simulink model "RTForwardVehicleSensorFusionHost"  (R2022a)
settings: Solver=FixedStepAuto  StartTime=0.0  StopTime=scenario.StopTime  RelTol=1e-3
PostLoadFcn:
  | helperSLForwardVehicleSensorFusionHostSetup
values from neighbouring files (symbols this model uses):
  camera = cameraParams(egoVehicle)    [helperSLForwardVehicleSensorFusionHostSetup.m]
  vehSim3D = repmat(     struct(         'Length', 0,         'RearOverhang', 0,         'InitialPos',[0 0 0],         'InitialRot',[0 0 0]),     numVehicles,1)    [helperSLForwardVehicleSensorFusionHostSetup.m]
undefined symbols (not defined in the file or in its folder): maxNumRadarDets, maxNumTracks, maxNumVisionDets, Ts
libraries: drivingscenarioandsensors x8, sim3dautolib x6, slrealtimeiplib x3, slrealtimeutilitieslib x3, simulink x1, sim3dprobsensorlib x1, sim3dlib x1, drivingsim3d x1
CloseFcn:
  | helperSLForwardVehicleSensorFusionHostCleanUp
settings Model: SILPILSystemUnderTest=refmodels  PacingRate=0.050000  Creator=The MathWorks, Inc.  LastModifiedBy=The MathWorks, Inc.
settings SolverCC: AlgebraicLoopSolver=TrustRegion  MaxZcPerStep=1
settings DataIOCC: SaveOutput=off  SaveTime=off  ReturnWorkspaceOutputs=off
settings OptimizationCC: ZeroExternalMemoryAtStartup=off  ZeroInternalMemoryAtStartup=off
settings DebuggingCC: ParameterPrecisionLossMsg=none  UnconnectedInputMsg=warning  UnconnectedOutputMsg=warning  UnconnectedLineMsg=warning  PregeneratedLibrarySubsystemCodeDiagnostic=none  SFMachineParentedDataDiag=warning  ArithmeticOperatorsInVariantConditions=warning
settings HardwareCC: ProdLongLongMode=on
settings SFSimCC: SimUseLocalCustomCode=off  SimTargetLang=C++
settings RTWCC: RTWUseLocalCustomCode=off  TargetLang=C++  DLArmComputeVersion=19.05
settings GRTTargetCC: TargetLangStandard=C++03 (ISO)  CodeInterfacePackaging=C++ class  RTWCAPISignals=on
settings ConfigComp: CovScope=ReferencedModels  CovIncludeTopModel=off

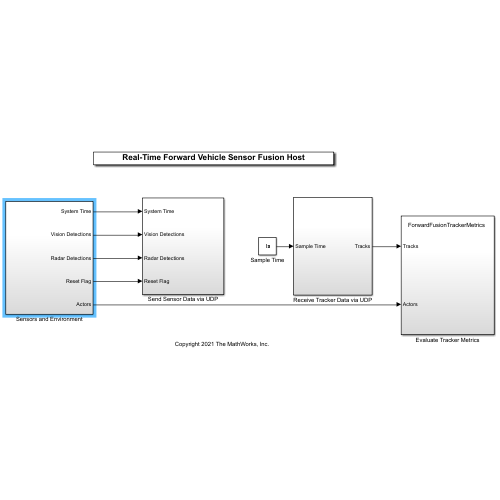
[thumbnail: Simulink's stored preview of the top-level diagram]
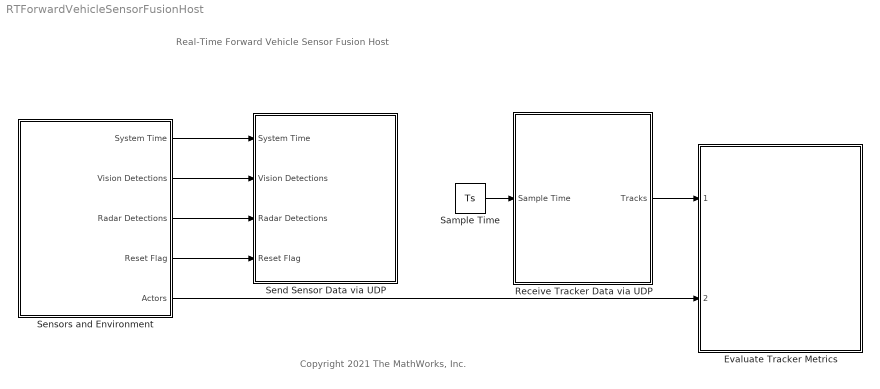
== system RTForwardVehicleSensorFusionHost ==
  note: Real-Time Forward Vehicle Sensor Fusion Host
  note: Copyright 2021 The MathWorks, Inc.
  Evaluate Tracker Metrics : Subsystem  ReferencedSubsystem=ForwardFusionTrackerMetrics
  Receive Tracker Data via UDP : Subsystem
  Sample Time : Constant  Value=Ts  SampleTime=Ts
  Send Sensor Data via UDP : Subsystem
  Sensors and Environment : Subsystem  VariantControl=1
  wires:
  Sensors and Environment/5(Actors) -> Evaluate Tracker Metrics/2
  Receive Tracker Data via UDP/1(Tracks) -> Evaluate Tracker Metrics/1
  Sensors and Environment/2(Vision Detections) -> Send Sensor Data via UDP/2(Vision Detections)
  Sensors and Environment/3(Radar Detections) -> Send Sensor Data via UDP/3(Radar Detections)
  Sensors and Environment/1(System Time) -> Send Sensor Data via UDP/1(System Time)
  Sample Time/1 -> Receive Tracker Data via UDP/1(Sample Time)
  Sensors and Environment/4(Reset Flag) -> Send Sensor Data via UDP/4(Reset Flag)

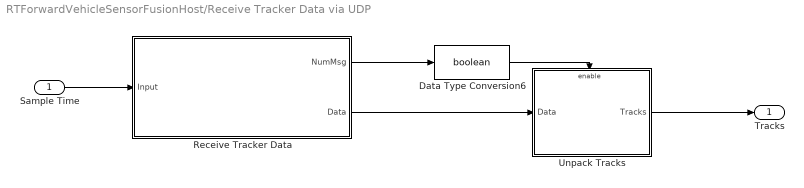
== system RTForwardVehicleSensorFusionHost/Receive Tracker Data via UDP ==
  Sample Time : Inport
  Data Type Conversion6 : DataTypeConversion  OutDataTypeStr=boolean  SaturateOnIntegerOverflow=off  RndMeth=Floor
  Receive Tracker Data : Subsystem
  Unpack Tracks : Subsystem
  Tracks : Outport
  wires:
  Data Type Conversion6/1 -> Unpack Tracks/Enable
  Receive Tracker Data/1(NumMsg) -> Data Type Conversion6/1
  Unpack Tracks/1(Tracks) -> Tracks/1
  Receive Tracker Data/2(Data) -> Unpack Tracks/1(Data)
  Sample Time/1 -> Receive Tracker Data/1(Input)

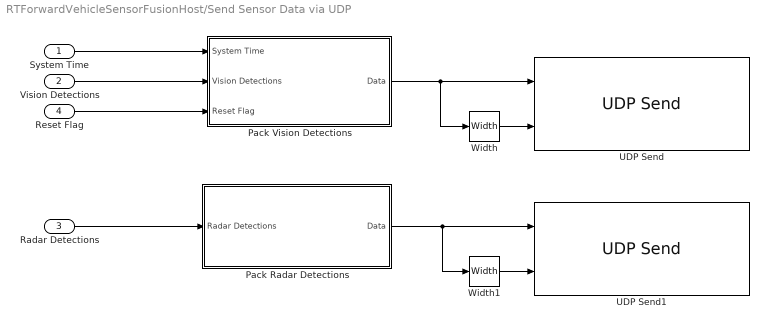
== system RTForwardVehicleSensorFusionHost/Send Sensor Data via UDP ==
  System Time : Inport
  Vision Detections : Inport  Port=2
  Radar Detections : Inport  Port=3
  Reset Flag : Inport  Port=4
  Pack Radar Detections : Subsystem
  Pack Vision Detections : Subsystem
  UDP Send : slrealtimeiplib/UDP Send  useHostTargetConn=on  toAddress=10.1.10.17  toPort=8001  sampleTime=-1  enableMessage=off  ipAddress=10.1.10.16  localPort=-1
      settings: SourceProductBaseCode=XP
  UDP Send1 : slrealtimeiplib/UDP Send  useHostTargetConn=on  toAddress=10.1.10.17  toPort=8002  sampleTime=-1  enableMessage=off  ipAddress=10.1.10.16  localPort=-1
      settings: SourceProductBaseCode=XP
  Width : Width
  Width1 : Width
  wires:
  Width/1 -> UDP Send/2
  Width1/1 -> UDP Send1/2
  Pack Vision Detections/1(Data) -> Width/1, UDP Send/1
  System Time/1 -> Pack Vision Detections/1(System Time)
  Vision Detections/1 -> Pack Vision Detections/2(Vision Detections)
  Reset Flag/1 -> Pack Vision Detections/3(Reset Flag)
  Pack Radar Detections/1(Data) -> Width1/1, UDP Send1/1
  Radar Detections/1 -> Pack Radar Detections/1(Radar Detections)

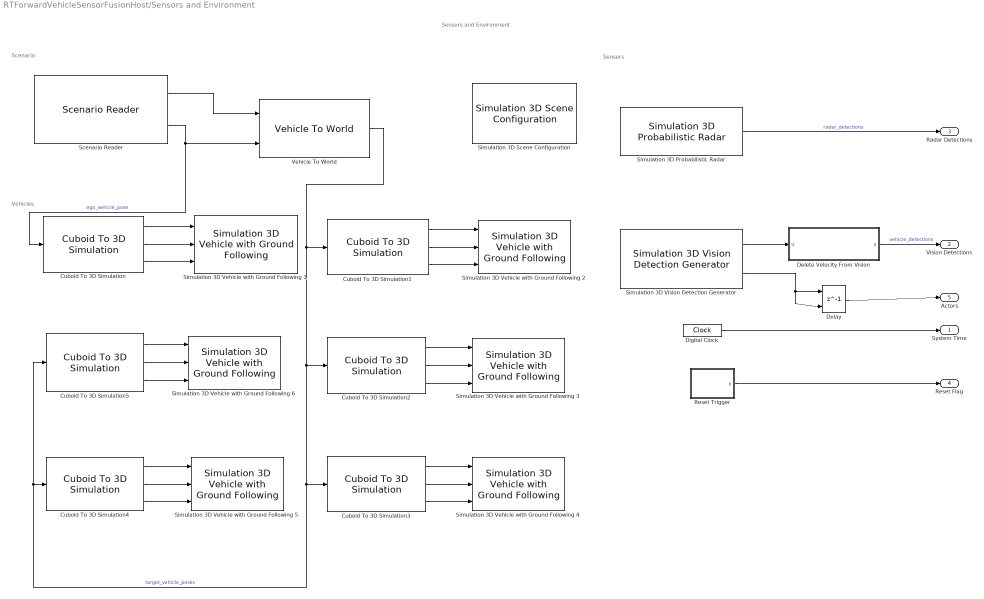
== system RTForwardVehicleSensorFusionHost/Sensors and Environment ==
  note: Sensors
  note: Sensors and Environment
  note: Scenario
  note: Vehicles
  Cuboid To 3D Simulation : drivingscenarioandsensors/Cuboid To 3D Simulation  SpecifyActorID=off  ActorIDToConvert=1  SimulateUsing=Interpreted execution
      settings: SourceProductBaseCode=DR
  Cuboid To 3D Simulation1 : drivingscenarioandsensors/Cuboid To 3D Simulation  SpecifyActorID=on  ActorIDToConvert=2  SimulateUsing=Interpreted execution
      settings: SourceProductBaseCode=DR
  Cuboid To 3D Simulation2 : drivingscenarioandsensors/Cuboid To 3D Simulation  SpecifyActorID=on  ActorIDToConvert=3  SimulateUsing=Interpreted execution
      settings: SourceProductBaseCode=DR
  Cuboid To 3D Simulation3 : drivingscenarioandsensors/Cuboid To 3D Simulation  SpecifyActorID=on  ActorIDToConvert=4  SimulateUsing=Interpreted execution
      settings: SourceProductBaseCode=DR
  Cuboid To 3D Simulation4 : drivingscenarioandsensors/Cuboid To 3D Simulation  SpecifyActorID=on  ActorIDToConvert=5  SimulateUsing=Interpreted execution
      settings: SourceProductBaseCode=DR
  Cuboid To 3D Simulation5 : drivingscenarioandsensors/Cuboid To 3D Simulation  SpecifyActorID=on  ActorIDToConvert=6  SimulateUsing=Interpreted execution
      settings: SourceProductBaseCode=DR
  Delay : Delay  DelayLength=1  InitialConditionSource=Input port
      settings: InputPortMap=u0,p4
  "Delete Velocity From Vision " : MATLAB Function  TreatAsAtomicUnit=on  mask(Pack vision detections){structInit=Simulink.Bus.createMATLABStruct('BusVision'), measurementNoise=camera.MeasurementNoise}
      mask prompts: structInit "Output struct"; measurementNoise "Measurement noise"
      mask help: Packs vision detections to match bus used by vision processing algorithm. This includes replacing the measurement noise and disabling the velocity measurement.
  Digital Clock : DigitalClock  SampleTime=Ts
  Reset Trigger : MATLAB Function  TreatAsAtomicUnit=on
  Scenario Reader : drivingscenarioandsensors/Scenario Reader  ScenarioSource=From workspace  ScenarioFileName=dblLaneChangeDrivingScenario.mat  ScenarioVariableName=scenario  OutputCoordinateSystem=Vehicle coordinates  EgoVehicleSource=Scenario  EgoVehicleActorID=1  OrientVehiclesOnRoad=off  OutputEgoVehiclePose=on  OutputEgoVehicleState=off  SampleTime=0.1  LaneBoundaryOutput=None  LaneBoundaryDistance=0:0.5:70  LaneBoundaryLocation=Center of lane markings  BusNameSource=Auto  BusName=BusActors  BusNumActorsSource=Scenario  BusNumActors=100  BusName2Source=Auto  BusName2=BusLaneBoundaries  BusNumLaneBoundariesSource=Scenario  BusNumLaneBoundaries=10  BusName3Source=Auto  BusName3=BusEgoActor  BusName4Source=Auto  BusName4=BusEgoState  ShowCoordinateLabels=on  SimulateUsing=Interpreted execution
  Simulation 3D Probabilistic Radar : sim3dprobsensorlib/Simulation 3D Probabilistic Radar  Priority=1  sensorTag=Sim3dSensor2  sensorId=2  sensorName=Sim3dSensor2  vehTagList={'Scene Origin';'SimulinkVehicle1';'SimulinkVehicle2';'SimulinkVehicle3';'SimulinkVehicle4';'SimulinkVehicle5';'SimulinkVehicle6'}  vehTag=SimulinkVehicle1  mountLoc=Origin  offsetFlag=on  tmountOffset=radar.PositionSim3d  rmountOffset=radar.Rotation  AzimuthResolution=0.8  ElevationResolution=8  RangeResolution=1  RangeRateResolution=1  AzimuthBiasFraction=0.1  ElevationBiasFraction=0.1  RangeBiasFraction=0.05  RangeRateBiasFraction=0.05  FieldOfView=radar.FieldOfView  DetectionRange=radar.DetectionRanges  RangeRateLimits=[ -100, 100 ]  DetectionProbability=0.9  FalseAlarmRate=1e-6  ReferenceRange=100  ReferenceRCS=0  HasElevation=off  HasRangeRate=on  HasNoise=off  HasFalseAlarms=off  InitialSeedSource=Specify seed  InitialSeed=1  MaxNumDetections=50  DetectionCoordinates=Sensor spherical  SpecifyOutputBusName=off  BusName=BusSimulation3DRadarTruthSensor  SampleTime=-1  mountPoint=[2.424 0 0.8]  mountOrientation=[0 0 0]  aMode=3  ID=2
      settings: SourceProductBaseCode=VE,AE,DR,UV,VE
      settings: AttributesFormatString=|
      | -------------------------------------
      | FieldOfView = %<FieldOfView>
      | AzimuthResolution = %<AzimuthResolution>
      | DetectionCoordinates = %<DetectionCoordinates>
      | mountLoc = %<mountLoc>
      | tmountOffset = %<tmountOffset>
      | rmountOffset = %<rmountOffset>
      | Priority = %<Priority>
  Simulation 3D Scene Configuration : sim3dlib/Simulation 3D Scene Configuration  Priority=0  ProjectFormat=Default Scenes  SceneDesc=Curved road  ProjectName=/mathworks/devel/bat/BR2022ad/build/matlab/toolbox/shared/sim3d_projects/automotive_project/UE4/LinuxNoEditor/AutoVrtlEnv.sh  ScenePath=/Game/Maps/HwStrght  vehTagList={'Scene Origin';'SimulinkVehicle1';'SimulinkVehicle2';'SimulinkVehicle3';'SimulinkVehicle4';'SimulinkVehicle5';'SimulinkVehicle6'}  vehTag=SimulinkVehicle1  OpVisEn=off  Ts=0.1  EnableWindow=on  EnableRemoteAccess=off  EnableWeather=off  SunAltitude=40.0  SunAzimuth=90  clouds=10  wind=1  fog=0  rain=0  sensorTag=MainCamera1  sensorId=1  sensorName=MainCamera1  mountLoc=Origin  offsetFlag=off  tmountOffset=[0, 0, 0]  rmountOffset=[0, 0, 0]  HorizontalResolution=1280  VerticalResolution=720  HorizontalFOV=60  mountPoint=[0 0 0]  mountOrientation=[0 0 0]  aMode=3  ID=1
      settings: SourceProductBaseCode=VE,AE,DR,UV,VE
      settings: AttributesFormatString=|
      | -------------------------------------
      | SceneName = %<SceneDesc>
      | Priority = %<Priority>
  Simulation 3D Vehicle with Ground Following 1 : sim3dautolib/Simulation 3D Vehicle with Ground Following  Priority=-1  PassVehMesh=Sedan  MeshPath=/MathWorksSimulation/Vehicles/Muscle/Meshes/SK_MuscleCar.SK_MuscleCar  TrackWidth=1.9  WheelBase=3  WheelRadius=0.35  VehColor=Blue  InitialPos=vehSim3D(1).InitialPos  InitialRot=vehSim3D(1).InitialRot  ActorName=SimulinkVehicle1  SampleTime=-1  ActorType=SimulinkVehicle  ID=1  aMode=3  ActorTag=SimulinkVehicle1  CoordinateScheme=ISO  VehLightsControl=off  HeadlightColor=[ 1, 1, 1 ]  HighBeamIntensity=100000  LowBeamIntensity=60000  HighBeamConeAngle=70  LowBeamConeAngle=70  LeftHeadlightOrientation=[ 0, 0 ]  RightHeadlightOrientation=[ 0, 0 ]  BrakelightIntensity=500  ReverselightIntensity=500  SignallightIntensity=500  SignallightPeriod=1  SignalPulseWidth=50  TransformOutportEnabled=off
      settings: SourceProductBaseCode=VE,AE,DR,UV,VE
      settings: AttributesFormatString=|
      | --------------------------------------
      | ActorName = %<ActorName>
      | PassVehMesh = %<PassVehMesh>
      | VehColor = %<VehColor>
      | InitialPos = %<InitialPos>
      | InitialRot = %<InitialRot>
      | Priority = %<Priority>
  Simulation 3D Vehicle with Ground Following 2 : sim3dautolib/Simulation 3D Vehicle with Ground Following  Priority=-1  PassVehMesh=Sedan  MeshPath=/MathWorksSimulation/Vehicles/Muscle/Meshes/SK_MuscleCar.SK_MuscleCar  TrackWidth=1.9  WheelBase=3  WheelRadius=0.35  VehColor=Red  InitialPos=vehSim3D(2).InitialPos  InitialRot=vehSim3D(2).InitialRot  ActorName=SimulinkVehicle2  SampleTime=-1  ActorType=SimulinkVehicle  ID=2  aMode=3  ActorTag=SimulinkVehicle2  CoordinateScheme=ISO  VehLightsControl=off  HeadlightColor=[ 1, 1, 1 ]  HighBeamIntensity=100000  LowBeamIntensity=60000  HighBeamConeAngle=70  LowBeamConeAngle=70  LeftHeadlightOrientation=[ 0, 0 ]  RightHeadlightOrientation=[ 0, 0 ]  BrakelightIntensity=500  ReverselightIntensity=500  SignallightIntensity=500  SignallightPeriod=1  SignalPulseWidth=50  TransformOutportEnabled=off
      settings: SourceProductBaseCode=VE,AE,DR,UV,VE
      settings: AttributesFormatString=|
      | --------------------------------------
      | ActorName = %<ActorName>
      | PassVehMesh = %<PassVehMesh>
      | VehColor = %<VehColor>
      | InitialPos = %<InitialPos>
      | InitialRot = %<InitialRot>
      | Priority = %<Priority>
  Simulation 3D Vehicle with Ground Following 3 : sim3dautolib/Simulation 3D Vehicle with Ground Following  Priority=-1  PassVehMesh=Muscle car  MeshPath=/MathWorksSimulation/Vehicles/Muscle/Meshes/SK_MuscleCar.SK_MuscleCar  TrackWidth=1.9  WheelBase=3  WheelRadius=0.35  VehColor=Black  InitialPos=vehSim3D(3).InitialPos  InitialRot=vehSim3D(3).InitialRot  ActorName=SimulinkVehicle3  SampleTime=-1  ActorType=SimulinkVehicle  ID=3  aMode=3  ActorTag=SimulinkVehicle3  CoordinateScheme=ISO  VehLightsControl=off  HeadlightColor=[ 1, 1, 1 ]  HighBeamIntensity=100000  LowBeamIntensity=60000  HighBeamConeAngle=70  LowBeamConeAngle=70  LeftHeadlightOrientation=[ 0, 0 ]  RightHeadlightOrientation=[ 0, 0 ]  BrakelightIntensity=500  ReverselightIntensity=500  SignallightIntensity=500  SignallightPeriod=1  SignalPulseWidth=50  TransformOutportEnabled=off
      settings: SourceProductBaseCode=VE,AE,DR,UV,VE
      settings: AttributesFormatString=|
      | --------------------------------------
      | ActorName = %<ActorName>
      | PassVehMesh = %<PassVehMesh>
      | VehColor = %<VehColor>
      | InitialPos = %<InitialPos>
      | InitialRot = %<InitialRot>
      | Priority = %<Priority>
  Simulation 3D Vehicle with Ground Following 4 : sim3dautolib/Simulation 3D Vehicle with Ground Following  Priority=-1  PassVehMesh=Hatchback  MeshPath=/MathWorksSimulation/Vehicles/Muscle/Meshes/SK_MuscleCar.SK_MuscleCar  TrackWidth=1.9  WheelBase=3  WheelRadius=0.35  VehColor=Orange  InitialPos=vehSim3D(4).InitialPos  InitialRot=vehSim3D(4).InitialRot  ActorName=SimulinkVehicle4  SampleTime=-1  ActorType=SimulinkVehicle  ID=4  aMode=3  ActorTag=SimulinkVehicle4  CoordinateScheme=ISO  VehLightsControl=off  HeadlightColor=[ 1, 1, 1 ]  HighBeamIntensity=100000  LowBeamIntensity=60000  HighBeamConeAngle=70  LowBeamConeAngle=70  LeftHeadlightOrientation=[ 0, 0 ]  RightHeadlightOrientation=[ 0, 0 ]  BrakelightIntensity=500  ReverselightIntensity=500  SignallightIntensity=500  SignallightPeriod=1  SignalPulseWidth=50  TransformOutportEnabled=off
      settings: SourceProductBaseCode=VE,AE,DR,UV,VE
      settings: AttributesFormatString=|
      | --------------------------------------
      | ActorName = %<ActorName>
      | PassVehMesh = %<PassVehMesh>
      | VehColor = %<VehColor>
      | InitialPos = %<InitialPos>
      | InitialRot = %<InitialRot>
      | Priority = %<Priority>
  Simulation 3D Vehicle with Ground Following 5 : sim3dautolib/Simulation 3D Vehicle with Ground Following  Priority=-1  PassVehMesh=Small pickup truck  MeshPath=/MathWorksSimulation/Vehicles/Muscle/Meshes/SK_MuscleCar.SK_MuscleCar  TrackWidth=1.9  WheelBase=3  WheelRadius=0.35  VehColor=Green  InitialPos=vehSim3D(5).InitialPos  InitialRot=vehSim3D(5).InitialRot  ActorName=SimulinkVehicle5  SampleTime=-1  ActorType=SimulinkVehicle  ID=5  aMode=3  ActorTag=SimulinkVehicle5  CoordinateScheme=ISO  VehLightsControl=off  HeadlightColor=[ 1, 1, 1 ]  HighBeamIntensity=100000  LowBeamIntensity=60000  HighBeamConeAngle=70  LowBeamConeAngle=70  LeftHeadlightOrientation=[ 0, 0 ]  RightHeadlightOrientation=[ 0, 0 ]  BrakelightIntensity=500  ReverselightIntensity=500  SignallightIntensity=500  SignallightPeriod=1  SignalPulseWidth=50  TransformOutportEnabled=off
      settings: SourceProductBaseCode=VE,AE,DR,UV,VE
      settings: AttributesFormatString=|
      | --------------------------------------
      | ActorName = %<ActorName>
      | PassVehMesh = %<PassVehMesh>
      | VehColor = %<VehColor>
      | InitialPos = %<InitialPos>
      | InitialRot = %<InitialRot>
      | Priority = %<Priority>
  Simulation 3D Vehicle with Ground Following 6 : sim3dautolib/Simulation 3D Vehicle with Ground Following  Priority=-1  PassVehMesh=Sport utility vehicle  MeshPath=/MathWorksSimulation/Vehicles/Muscle/Meshes/SK_MuscleCar.SK_MuscleCar  TrackWidth=1.9  WheelBase=3  WheelRadius=0.35  VehColor=Blue  InitialPos=vehSim3D(6).InitialPos  InitialRot=vehSim3D(6).InitialRot  ActorName=SimulinkVehicle6  SampleTime=-1  ActorType=SimulinkVehicle  ID=6  aMode=3  ActorTag=SimulinkVehicle6  CoordinateScheme=ISO  VehLightsControl=off  HeadlightColor=[ 1, 1, 1 ]  HighBeamIntensity=100000  LowBeamIntensity=60000  HighBeamConeAngle=70  LowBeamConeAngle=70  LeftHeadlightOrientation=[ 0, 0 ]  RightHeadlightOrientation=[ 0, 0 ]  BrakelightIntensity=500  ReverselightIntensity=500  SignallightIntensity=500  SignallightPeriod=1  SignalPulseWidth=50  TransformOutportEnabled=off
      settings: SourceProductBaseCode=VE,AE,DR,UV,VE
      settings: AttributesFormatString=|
      | --------------------------------------
      | ActorName = %<ActorName>
      | PassVehMesh = %<PassVehMesh>
      | VehColor = %<VehColor>
      | InitialPos = %<InitialPos>
      | InitialRot = %<InitialRot>
      | Priority = %<Priority>
  Simulation 3D Vision Detection Generator : drivingsim3d/Simulation 3D Vision Detection Generator  Priority=1  sensorTag=Sim3dSensor255  sensorId=1  sensorName=Sim3dSensor1  vehTagList={'Scene Origin';'SimulinkVehicle1';'SimulinkVehicle2';'SimulinkVehicle3';'SimulinkVehicle4';'SimulinkVehicle5';'SimulinkVehicle6'}  vehTag=SimulinkVehicle1  mountLoc=Origin  offsetFlag=on  tmountOffset=camera.PositionSim3d  rmountOffset=camera.Rotation  DetectorOutput=Objects only  MaxNumDetections=20  MaxNumLanes=30  laneSampleDistances=0:0.5:9.5  BusNameSource=Property  BusName=BusObjectDetections  BusName2Source=Auto  BusName2=BusLaneDetections  MaxRange=camera.DetectionRanges(2)  BoundingBoxAccuracy=5  ProcessNoiseIntensity=5  MaxSpeed=50  MaxAllowedOcclusion=0.5  MinObjectImageSize=camera.MinObjectImageSize  DetectionProbability=0.9  FalsePositivesPerImage=0  MinLaneImageSize=[ 20, 3 ]  LaneBoundaryAccuracy=3  HasNoise=off  InitialSeedSource=Specify seed  InitialSeed=1  uniqueActorIdentifier=[]  actorClassInteger=0  cuboidLength=4.7  cuboidWidth=1.8  cuboidHeight=1.4  rotationalCenter={[-1.35, 0, 0]}  focalLength=camera.FocalLength  opticalCenter=camera.PrincipalPoint  imageSize=camera.ImageSize  radialDistortionCoefficients=[0, 0]  tangentialDistortionCoefficients=[0, 0]  cameraAxisSkew=0  actorTruthOutportEnabled=on  laneTruthOutportEnabled=off  SampleTime=-1  checkedSampleTime=0.1  mountPoint=[0.57 0 1.2]  mountOrientation=[0 0 0]  aMode=3  ID=1
      settings: SourceProductBaseCode=DR
  Vehicle To World : drivingscenarioandsensors/Vehicle To World  BusNameSource=Auto  BusName=BusVehicleToWorldActors  SimulateUsing=Interpreted execution
      settings: SourceProductBaseCode=DR
  System Time : Outport  VectorParamsAs1DForOutWhenUnconnected=off
  Vision Detections : Outport  Port=2  OutDataTypeStr=Bus:BusVision
  Radar Detections : Outport  Port=3
  Reset Flag : Outport  Port=4
  Actors : Outport  Port=5
  wires:
  Cuboid To 3D Simulation/1 -> Simulation 3D Vehicle with Ground Following 1/1
  Cuboid To 3D Simulation/3 -> Simulation 3D Vehicle with Ground Following 1/3
  Cuboid To 3D Simulation/2 -> Simulation 3D Vehicle with Ground Following 1/2
  Cuboid To 3D Simulation1/2 -> Simulation 3D Vehicle with Ground Following 2/2
  Cuboid To 3D Simulation1/3 -> Simulation 3D Vehicle with Ground Following 2/3
  Cuboid To 3D Simulation1/1 -> Simulation 3D Vehicle with Ground Following 2/1
  Scenario Reader/1 -> Vehicle To World/1
  Scenario Reader/2 -> Cuboid To 3D Simulation/1, Vehicle To World/2  "ego_vehicle_pose"
  Simulation 3D Probabilistic Radar/1 -> Radar Detections/1  "radar_detections"
  Vehicle To World/1 -> Cuboid To 3D Simulation1/1, Cuboid To 3D Simulation2/1, Cuboid To 3D Simulation3/1, Cuboid To 3D Simulation5/1, Cuboid To 3D Simulation4/1  "target_vehicle_poses"
  Cuboid To 3D Simulation2/2 -> Simulation 3D Vehicle with Ground Following 3/2
  Cuboid To 3D Simulation2/1 -> Simulation 3D Vehicle with Ground Following 3/1
  Cuboid To 3D Simulation2/3 -> Simulation 3D Vehicle with Ground Following 3/3
  Cuboid To 3D Simulation3/2 -> Simulation 3D Vehicle with Ground Following 4/2
  Cuboid To 3D Simulation3/1 -> Simulation 3D Vehicle with Ground Following 4/1
  Cuboid To 3D Simulation3/3 -> Simulation 3D Vehicle with Ground Following 4/3
  Cuboid To 3D Simulation4/2 -> Simulation 3D Vehicle with Ground Following 5/2
  Cuboid To 3D Simulation4/1 -> Simulation 3D Vehicle with Ground Following 5/1
  Cuboid To 3D Simulation4/3 -> Simulation 3D Vehicle with Ground Following 5/3
  Cuboid To 3D Simulation5/2 -> Simulation 3D Vehicle with Ground Following 6/2
  Cuboid To 3D Simulation5/1 -> Simulation 3D Vehicle with Ground Following 6/1
  Cuboid To 3D Simulation5/3 -> Simulation 3D Vehicle with Ground Following 6/3
  Digital Clock/1 -> System Time/1
  Simulation 3D Vision Detection Generator/1 -> "Delete Velocity From Vision "/1(u)
  "Delete Velocity From Vision "/1(y) -> Vision Detections/1  "vehicle_detections"
  Simulation 3D Vision Detection Generator/2 -> Delay/2, Delay/1
  Reset Trigger/1(y) -> Reset Flag/1
  Delay/1 -> Actors/1

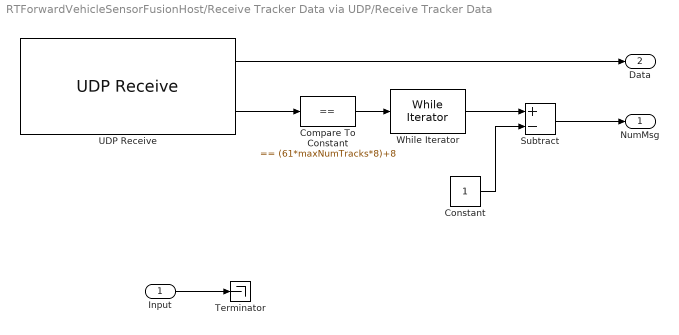
== system RTForwardVehicleSensorFusionHost/Receive Tracker Data via UDP/Receive Tracker Data ==
  Input : Inport
  Compare To Constant : simulink/Logic and Bit Operations/Compare To Constant  relop===  const=(61*maxNumTracks*8)+8  OutDataTypeStr=boolean
  Constant : Constant
  Subtract : Sum  Inputs=+-
  Terminator : Terminator
  UDP Receive : slrealtimeiplib/UDP Receive  useHostTargetConn=on  ipAddress=10.1.10.16  localPort=8021  rcvWidth=(61*maxNumTracks*8)+8  rcvFmAny=off  fmAddress=10.1.10.17  sampleTime=-1  enableMessage=off  maxPackets=1
      settings: SourceProductBaseCode=XP
  While Iterator : WhileIterator  WhileBlockType=do-while  ResetStates=reset  ShowIterationPort=on
  NumMsg : Outport
  Data : Outport  Port=2
  wires:
  Input/1 -> Terminator/1
  UDP Receive/2 -> Compare To Constant/1
  Subtract/1 -> NumMsg/1
  UDP Receive/1 -> Data/1
  Compare To Constant/1 -> While Iterator/1
  Constant/1 -> Subtract/2
  While Iterator/1 -> Subtract/1

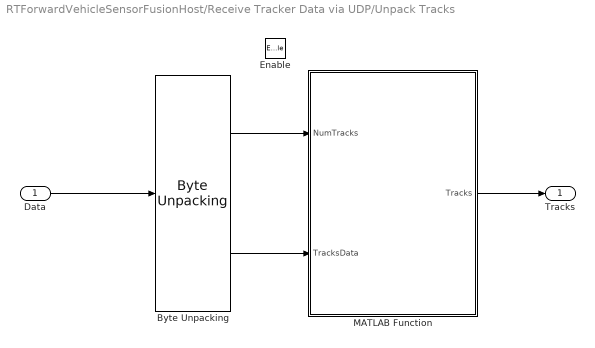
== system RTForwardVehicleSensorFusionHost/Receive Tracker Data via UDP/Unpack Tracks ==
  Data : Inport
  Enable : EnablePort
  "Byte Unpacking " : slrealtimeutilitieslib/Byte Unpacking  MaskUnpackedDataTypes={'double',['double']}  MaskUnpackedDataSizes={[1],[61*maxNumTracks]}  MaskAlignment=1
      settings: SourceProductBaseCode=XP
  "MATLAB Function " : MATLAB Function  TreatAsAtomicUnit=on  mask{structObj=Simulink.Bus.createMATLABStruct('BusTrackerJPDA');, maxNumTracks=maxNumTracks}
      mask prompts: structObj "Output struct"
  Tracks : Outport
  wires:
  "Byte Unpacking "/1 -> "MATLAB Function "/1(NumTracks)
  Data/1 -> "Byte Unpacking "/1
  "MATLAB Function "/1(Tracks) -> Tracks/1
  "Byte Unpacking "/2 -> "MATLAB Function "/2(TracksData)

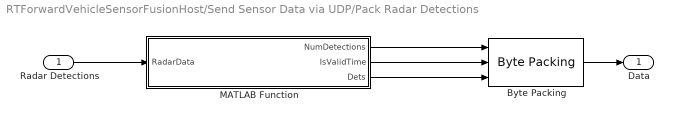
== system RTForwardVehicleSensorFusionHost/Send Sensor Data via UDP/Pack Radar Detections ==
  Radar Detections : Inport
  Byte Packing : slrealtimeutilitieslib/Byte Packing  MaskPackedDataType=uint8  MaskUnpackedDataTypes={'double', 'boolean', ['double']}  MaskAlignment=1
  MATLAB Function : MATLAB Function  TreatAsAtomicUnit=on  mask{maxNumDets=maxNumRadarDets}
  Data : Outport
  wires:
  MATLAB Function/3(Dets) -> Byte Packing/3
  MATLAB Function/2(IsValidTime) -> Byte Packing/2
  Byte Packing/1 -> Data/1
  MATLAB Function/1(NumDetections) -> Byte Packing/1
  Radar Detections/1 -> MATLAB Function/1(RadarData)

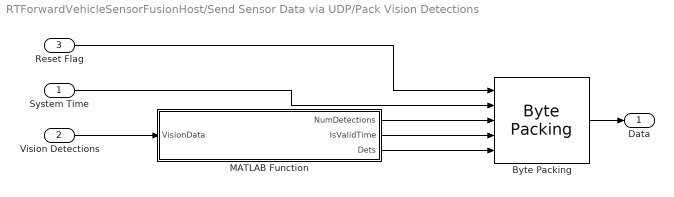
== system RTForwardVehicleSensorFusionHost/Send Sensor Data via UDP/Pack Vision Detections ==
  System Time : Inport
  Vision Detections : Inport  Port=2
  Reset Flag : Inport  Port=3
  Byte Packing : slrealtimeutilitieslib/Byte Packing  MaskPackedDataType=uint8  MaskUnpackedDataTypes={'double','double','double', 'boolean', ['double']}  MaskAlignment=1
  MATLAB Function : MATLAB Function  TreatAsAtomicUnit=on  mask{maxNumDets=maxNumVisionDets}
  Data : Outport
  wires:
  MATLAB Function/3(Dets) -> Byte Packing/5
  System Time/1 -> Byte Packing/2
  MATLAB Function/1(NumDetections) -> Byte Packing/3
  Byte Packing/1 -> Data/1
  MATLAB Function/2(IsValidTime) -> Byte Packing/4
  Vision Detections/1 -> MATLAB Function/1(VisionData)
  Reset Flag/1 -> Byte Packing/1

== matlab function RTForwardVehicleSensorFusionHost/Send Sensor Data via UDP/Pack Vision Detections/MATLAB Function ==
  data: VisionData input Bus: BusVision; NumDetections output; IsValidTime output; Dets output; maxNumDets parameter
function [NumDetections, IsValidTime, Dets] = busVisionToUdpData(VisionData, maxNumDets)
% busVisionToUdpData function converts the vision detections data structure
% (BusVision) into UDP data.

% Define data vector to store detections data.
Dets = zeros(1, maxNumDets*30, 'double');

% Assign number of detections to the output variable.
NumDetections = VisionData.NumDetections;

% Assign valid time flag to the output variable.
IsValidTime   = VisionData.IsValidTime;

% Get sizes of structure elements into a vector.
sizesVector = [numel(VisionData.Detections(1).Time), ...
               numel(VisionData.Detections(1).Measurement), ...
               numel(VisionData.Detections(1).MeasurementNoise), ...
               numel(VisionData.Detections(1).SensorIndex), ...
               numel(VisionData.Detections(1).ObjectClassID), ...
               numel(VisionData.Detections(1).MeasurementParameters.Frame), ...
               numel(VisionData.Detections(1).MeasurementParameters.OriginPosition), ...
               numel(VisionData.Detections(1).MeasurementParameters.Orientation), ...
               numel(VisionData.Detections(1).MeasurementParameters.HasVelocity), ...
               numel(VisionData.Detections(1).ObjectAttributes.TargetIndex)];

% Assign detections data to data vector.
k = 1;
for i=1:maxNumDets
    Dets(k) = VisionData.Detections(i).Time;k=k+sizesVector(1);
    Dets(k:k+sizesVector(2)-1) = VisionData.Detections(i).Measurement;k=k+sizesVector(2);
    Dets(k:k+sizesVector(3)-1) = VisionData.Detections(i).MeasurementNoise(:);k=k+sizesVector(3);
    Dets(k) = VisionData.Detections(i).SensorIndex;k=k+sizesVector(4);
    Dets(k) = VisionData.Detections(i).ObjectClassID;k=k+sizesVector(5);
    Dets(k) = VisionData.Detections(i).MeasurementParameters.Frame;k=k+sizesVector(6);
    Dets(k:k+sizesVector(7)-1) = VisionData.Detections(i).MeasurementParameters.OriginPosition;k=k+sizesVector(7);
    Dets(k:k+sizesVector(8)-1) = VisionData.Detections(i).MeasurementParameters.Orientation;k=k+sizesVector(8);
    Dets(k) = VisionData.Detections(i).MeasurementParameters.HasVelocity;k=k+sizesVector(9);
    Dets(k) = VisionData.Detections(i).ObjectAttributes.TargetIndex;k=k+sizesVector(10);
end

== matlab function RTForwardVehicleSensorFusionHost/Sensors and Environment/Delete Velocity From Vision  ==
  data: u input; y output Bus: BusVision; structInit parameter; measurementNoise parameter
function y = deleteVelocityFromVision(u,structInit,measurementNoise)

y = structInit;
y.NumDetections = u.NumDetections;
y.IsValidTime = u.IsValidTime;
for n = 1:u.NumDetections
    y.Detections(n).Time = u.Detections(n).Time;
    y.Detections(n).Measurement = u.Detections(n).Measurement(1:3);
    y.Detections(n).MeasurementNoise = measurementNoise;
    y.Detections(n).SensorIndex = u.Detections(n).SensorIndex;
    y.Detections(n).ObjectClassID = u.Detections(n).ObjectClassID;
    y.Detections(n).ObjectAttributes = u.Detections(n).ObjectAttributes;
    y.Detections(n).MeasurementParameters = u.Detections(n).MeasurementParameters;
    y.Detections(n).MeasurementParameters.HasVelocity = false;
end

== matlab function RTForwardVehicleSensorFusionHost/Send Sensor Data via UDP/Pack Radar Detections/MATLAB Function ==
  data: RadarData input Bus: BusRadar; NumDetections output; IsValidTime output; Dets output; maxNumDets parameter
function [NumDetections, IsValidTime, Dets] = packRadarData(RadarData, maxNumDets)
% busRadarToUdpData function converts the radar detections data structure
% (BusRadar) into UDP data.

% Define data vector to store detections data.
Dets = zeros(1, 32*maxNumDets, 'double');

% Assign number of detections to the output variable.
NumDetections = RadarData.NumDetections;

% Assign valid time flag to the output variable.
IsValidTime   = RadarData.IsValidTime;

% Get sizes of structure elements into a vector.
sizesVector = [numel(RadarData.Detections(1).Time), ...
               numel(RadarData.Detections(1).Measurement), ...
               numel(RadarData.Detections(1).MeasurementNoise(:)), ...
               numel(RadarData.Detections(1).SensorIndex), ...
               numel(RadarData.Detections(1).ObjectClassID), ...
               numel(RadarData.Detections(1).MeasurementParameters.Frame), ...
               numel(RadarData.Detections(1).MeasurementParameters.OriginPosition), ...
               numel(RadarData.Detections(1).MeasurementParameters.Orientation), ...
               numel(RadarData.Detections(1).MeasurementParameters.HasVelocity), ...
               numel(RadarData.Detections(1).MeasurementParameters.HasElevation), ...
               numel(RadarData.Detections(1).ObjectAttributes.TargetIndex), ...
               numel(RadarData.Detections(1).ObjectAttributes.SNR)];

% Assign detections data to data vector.
k = 1;
for i=1:maxNumDets
    Dets(k) = RadarData.Detections(i).Time;k=k+sizesVector(1);
    Dets(k:k+sizesVector(2)-1) = RadarData.Detections(i).Measurement;k=k+sizesVector(2);
    Dets(k:k+sizesVector(3)-1) = RadarData.Detections(i).MeasurementNoise(:);k=k+sizesVector(3);
    Dets(k) = RadarData.Detections(i).SensorIndex;k=k+sizesVector(4);
    Dets(k) = RadarData.Detections(i).ObjectClassID;k=k+sizesVector(5);
    Dets(k) = RadarData.Detections(i).MeasurementParameters.Frame;k=k+sizesVector(6);
    Dets(k:k+sizesVector(7)-1) = RadarData.Detections(i).MeasurementParameters.OriginPosition;k=k+sizesVector(7);
    Dets(k:k+sizesVector(8)-1) = RadarData.Detections(i).MeasurementParameters.Orientation;k=k+sizesVector(8);
    Dets(k) = RadarData.Detections(i).MeasurementParameters.HasVelocity;k=k+sizesVector(9);
    Dets(k) = RadarData.Detections(i).MeasurementParameters.HasElevation;k=k+sizesVector(10);
    Dets(k) = RadarData.Detections(i).ObjectAttributes.TargetIndex;k=k+sizesVector(11);
    Dets(k) = RadarData.Detections(i).ObjectAttributes.SNR;k=k+sizesVector(12);
end

== matlab function RTForwardVehicleSensorFusionHost/Receive Tracker Data via UDP/Unpack Tracks/MATLAB Function  ==
  data: NumTracks input; Tracks output Bus: BusTrackerJPDA; TracksData input; structObj parameter; maxNumTracks parameter
function Tracks  = udpDataToBusTrackerJPDA(NumTracks, TracksData, ...
                                               structObj, maxNumTracks)
% udpDataToBusTrackerJPDA function fill up the tracks data structure
% (BusTrackerJPDA) with received UDP data.

% Assign tracks structure object to the output variable.
Tracks = structObj;

% Assign number of tracks value to the structure object.
if NumTracks > maxNumTracks
    Tracks.NumTracks = maxNumTracks;
else
    Tracks.NumTracks = NumTracks;
end

% Get sizes of structure elements into a vector.
sizesVector = [numel(Tracks.Tracks(1).TrackID),...
    numel(Tracks.Tracks(1).BranchID),...
    numel(Tracks.Tracks(1).SourceIndex),...
    numel(Tracks.Tracks(1).UpdateTime),...
    numel(Tracks.Tracks(1).Age),...
    numel(Tracks.Tracks(1).State),...
    numel(Tracks.Tracks(1).StateCovariance),...
    numel(Tracks.Tracks(1).ObjectClassID),...
    numel(Tracks.Tracks(1).TrackLogic),...
    numel(Tracks.Tracks(1).TrackLogicState),...
    numel(Tracks.Tracks(1).IsConfirmed),...
    numel(Tracks.Tracks(1).IsCoasted),...
    numel(Tracks.Tracks(1).IsSelfReported),...
    numel(Tracks.Tracks(1).ObjectAttributes(1).TargetIndex),...
    numel(Tracks.Tracks(1).ObjectAttributes(1).SNR),...
    numel(Tracks.Tracks(1).ObjectAttributes(2).TargetIndex),...
    numel(Tracks.Tracks(1).ObjectAttributes(2).SNR)];

% Fill up the structure object with received UDP data vector.
k = 1;
for i=1:NumTracks
    Tracks.Tracks(i).TrackID = uint32(TracksData(k));k=k+sizesVector(1);
    Tracks.Tracks(i).BranchID = uint32(TracksData(k));k=k+sizesVector(2);
    Tracks.Tracks(i).SourceIndex = uint32(TracksData(k));k=k+sizesVector(3);
    Tracks.Tracks(i).UpdateTime = TracksData(k);k=k+sizesVector(4);
    Tracks.Tracks(i).Age = uint32(TracksData(k));k=k+sizesVector(5);
    Tracks.Tracks(i).State = reshape(TracksData(k:k+sizesVector(6)-1), [6 1]);k=k+sizesVector(6);
    Tracks.Tracks(i).StateCovariance(:) = reshape(TracksData(k:k+sizesVector(7)-1), [6 6]);k=k+sizesVector(7);
    Tracks.Tracks(i).ObjectClassID = TracksData(k);k=k+sizesVector(8);
    Tracks.Tracks(i).TrackLogic = trackLogicType(TracksData(k));k=k+sizesVector(9);
    Tracks.Tracks(i).TrackLogicState(:) = boolean(reshape(TracksData(k:k+sizesVector(10)-1), [1 5]));k=k+sizesVector(10);
    Tracks.Tracks(i).IsConfirmed = boolean(TracksData(k));k=k+sizesVector(11);
    Tracks.Tracks(i).IsCoasted = boolean(TracksData(k));k=k+sizesVector(12);
    Tracks.Tracks(i).IsSelfReported = boolean(TracksData(k));k=k+sizesVector(13);
    Tracks.Tracks(i).ObjectAttributes(1).TargetIndex = TracksData(k);k=k+sizesVector(14);
    Tracks.Tracks(i).ObjectAttributes(1).SNR = TracksData(k);k=k+sizesVector(15);
    Tracks.Tracks(i).ObjectAttributes(2).TargetIndex = TracksData(k);k=k+sizesVector(16);
    Tracks.Tracks(i).ObjectAttributes(2).SNR = TracksData(k);k=k+sizesVector(17);
end

end

== matlab function RTForwardVehicleSensorFusionHost/Sensors and Environment/Reset Trigger ==
  data: y output
function y = resetFlagGen

persistent isStarted;

if isempty(isStarted)
    y = 1;
    isStarted = 1;
else
    y = 0;
end
